simulink model "Startbrenner_Funktionsblock"  (R2019b)
settings: Solver=VariableStepAuto  StartTime=0.0  StopTime=3000  RelTol=1e-3
values from neighbouring files (symbols this model uses):
  A = double(subs(subs(subs( jacobian(dx_dt,vec_x), vec_x, x_AP), vec_e, e_AP), vec_u, u_AP))    [Modellbildung_Startbrenner.m]
  B = double(subs(subs(subs( jacobian(dx_dt,vec_u), vec_x, x_AP), vec_e, e_AP), vec_u, u_AP))    [Modellbildung_Startbrenner.m]
  C = [1,0,0;0,1,0]    [Modellbildung_Startbrenner.m]
  E = double(subs(subs(subs( jacobian(dx_dt,vec_e), vec_x, x_AP), vec_e, e_AP), vec_u, u_AP))    [Modellbildung_Startbrenner.m]
  e_AP = [T_bg_in ; T_wt_in ; T_u]    [Modellbildung_Startbrenner.m]
  K = place(A,B,lambda_w)    [Modellbildung_Startbrenner.m]
  S_v = inv(C*(inv(-A+B*K))*B)    [Modellbildung_Startbrenner.m]
  T_Ini = [ 293.15  ; 293.15 ; 293.15  ]    [Modellbildung_Startbrenner.m]
  T_Ini_Lin = T_Ini - x_AP    [Modellbildung_Startbrenner.m]
  u_AP = [ m_sbg ; m_sair ]    [Modellbildung_Startbrenner.m]
  vec_par = zeros(17,1)    [Modellbildung_Startbrenner.m]
  vec_z = vec_T + e_AP    [Modellbildung_Startbrenner.m]
  w = [1200; 1000]    [Modellbildung_Startbrenner.m]
  x_AP = [double(x_AP_berechnet.x1) ; double(x_AP_berechnet.x2) ; double(x_AP_berechnet.x3)]    [Modellbildung_Startbrenner.m]
  y_AP = [double(x_AP_berechnet.x1) ; double(x_AP_berechnet.x2) ]    [Modellbildung_Startbrenner.m]
libraries: simulink x2
settings Model: Creator=mh981  LastModifiedBy=michael
settings DataIOCC: ReturnWorkspaceOutputs=off
settings DebuggingCC: ArithmeticOperatorsInVariantConditions=warning
settings SFSimCC: CustomCodeUndefinedFunction=UseInterfaceOnly

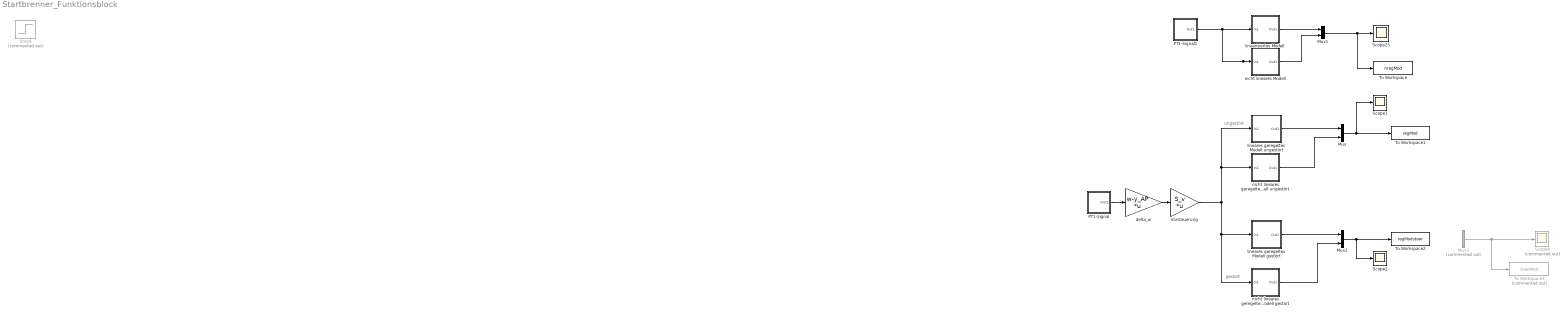
== system Startbrenner_Funktionsblock ==
  note: ungestört
  note: gestört
  Mux : Mux  Inputs=2
  Mux1 : Mux  Inputs=2
  Mux2 : Mux  Inputs=2
  Mux3 : Mux  Commented=on  Inputs=2
  PT1-Signal : Subsystem
  PT1-Signal1 : Subsystem
  Scope1 : Scope
  Scope2 : Scope
  Scope25 : Scope
  Scope4 : Scope  Commented=on
  Step4 : Step  Commented=on  Time=0  Before=u_AP  After=u_AP  SampleTime=0
  To Workspace : ToWorkspace  VariableName=nregMod  SaveFormat=Structure With Time  SampleTime=-1
  To Workspace1 : ToWorkspace  VariableName=regMod  SaveFormat=Structure With Time  SampleTime=-1
  To Workspace2 : ToWorkspace  VariableName=regModstoer  SaveFormat=Structure With Time  SampleTime=-1
  To Workspace3 : ToWorkspace  Commented=on  VariableName=stoerMod  SaveFormat=Structure With Time  SampleTime=-1
  Vorsteuerung : Gain  Gain=S_v  Multiplication=Matrix(K*u)
  delta_w : Gain  Gain=w-y_AP  Multiplication=Matrix(K*u)
  lineares geregeltes Modell gestört : Subsystem
  lineares geregeltes Modell ungestört : Subsystem
  linearisiertes Modell : Subsystem
  nicht lineares Modell : Subsystem
  nicht lineares geregeltes Modell gestört : Subsystem
  nicht lineares geregeltes Modell ungestört : Subsystem
  wires:
  PT1-Signal/1(Out1) -> delta_w/1
  delta_w/1 -> Vorsteuerung/1
  linearisiertes Modell/1(Out1) -> Mux1/1
  PT1-Signal1/1(Out1) -> linearisiertes Modell/1(In1), nicht lineares Modell/1(In1)
  Vorsteuerung/1 -> nicht lineares geregeltes Modell gestört/1(In1), lineares geregeltes Modell gestört/1(In1), lineares geregeltes Modell ungestört/1(In1), nicht lineares geregeltes Modell ungestört/1(In1)
  nicht lineares geregeltes Modell ungestört/1(Out1) -> Mux/2
  lineares geregeltes Modell ungestört/1(Out1) -> Mux/1
  nicht lineares Modell/1(Out1) -> Mux1/2
  Mux/1 -> To Workspace1/1, Scope1/1
  Mux1/1 -> Scope25/1, To Workspace/1
  Mux2/1 -> Scope2/1, To Workspace2/1
  lineares geregeltes Modell gestört/1(Out1) -> Mux2/1
  nicht lineares geregeltes Modell gestört/1(Out1) -> Mux2/2
  Mux3/1 -> To Workspace3/1, Scope4/1

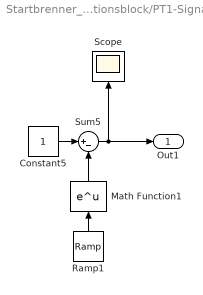
== system Startbrenner_Funktionsblock/PT1-Signal ==
  Constant5 : Constant
  Math Function1 : Math  SignedPower=off  SaturateOnIntegerOverflow=on
  Ramp1 : simulink/Sources/Ramp  slope=-1/t  start=0  InitialOutput=0
  Scope : Scope
  Sum5 : Sum  Inputs=|+-
  Out1 : Outport
  wires:
  Constant5/1 -> Sum5/1
  Math Function1/1 -> Sum5/2
  Ramp1/1 -> Math Function1/1
  Sum5/1 -> Out1/1, Scope/1

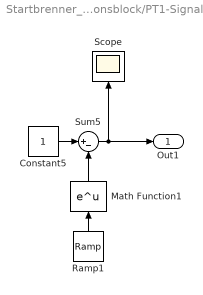
== system Startbrenner_Funktionsblock/PT1-Signal1 ==
  Constant5 : Constant
  Math Function1 : Math  SignedPower=off  SaturateOnIntegerOverflow=on
  Ramp1 : simulink/Sources/Ramp  slope=-1/t  start=0  InitialOutput=0
  Scope : Scope
  Sum5 : Sum  Inputs=|+-
  Out1 : Outport
  wires:
  Constant5/1 -> Sum5/1
  Math Function1/1 -> Sum5/2
  Ramp1/1 -> Math Function1/1
  Sum5/1 -> Out1/1, Scope/1

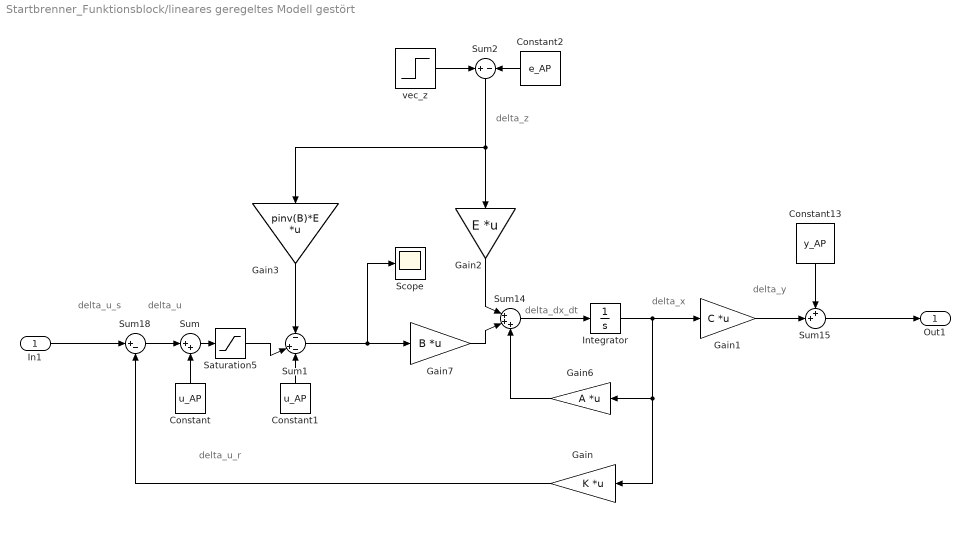
== system Startbrenner_Funktionsblock/lineares geregeltes Modell gestört ==
  note: delta_y
  note: delta_x
  note: delta_dx_dt
  note: delta_u_r
  note: delta_u
  note: delta_u_s
  note: delta_z
  In1 : Inport
  Constant : Constant  Value=u_AP
  Constant1 : Constant  Value=u_AP
  Constant13 : Constant  Value=y_AP
  Constant2 : Constant  Value=e_AP
  Gain : Gain  Gain=K  Multiplication=Matrix(K*u)
  Gain1 : Gain  Gain=C  Multiplication=Matrix(K*u)
  Gain2 : Gain  Gain=E  Multiplication=Matrix(K*u)
  Gain3 : Gain  Gain=pinv(B)*E  Multiplication=Matrix(K*u)
  Gain6 : Gain  Gain=A  Multiplication=Matrix(K*u)
  Gain7 : Gain  Gain=B  Multiplication=Matrix(K*u) (u vector)
  Integrator : Integrator  InitialCondition=T_Ini_Lin
  Saturation5 : Saturate  UpperLimit=2*u_AP  LowerLimit=0.1*u_AP
  Scope : Scope
  Sum : Sum  Inputs=|++
  Sum1 : Sum  Inputs=-|+-
  Sum14 : Sum  Inputs=|+++
  Sum15 : Sum  Inputs=++|
  Sum18 : Sum  Inputs=|+-
  Sum2 : Sum  Inputs=+|-
  vec_z : Step  Before=vec_z  After=vec_z  SampleTime=0
  Out1 : Outport
  wires:
  Gain1/1 -> Sum15/2
  Sum14/1 -> Integrator/1
  vec_z/1 -> Sum2/1
  Sum18/1 -> Sum/1
  Constant1/1 -> Sum1/3
  Gain/1 -> Sum18/2
  Gain2/1 -> Sum14/1
  Saturation5/1 -> Sum1/2
  Constant/1 -> Sum/2
  Sum15/1 -> Out1/1
  Gain6/1 -> Sum14/3
  Constant2/1 -> Sum2/2
  In1/1 -> Sum18/1
  Integrator/1 -> Gain6/1, Gain/1, Gain1/1
  Constant13/1 -> Sum15/1
  Sum/1 -> Saturation5/1
  Sum2/1 -> Gain3/1, Gain2/1
  Gain7/1 -> Sum14/2
  Gain3/1 -> Sum1/1
  Sum1/1 -> Scope/1, Gain7/1

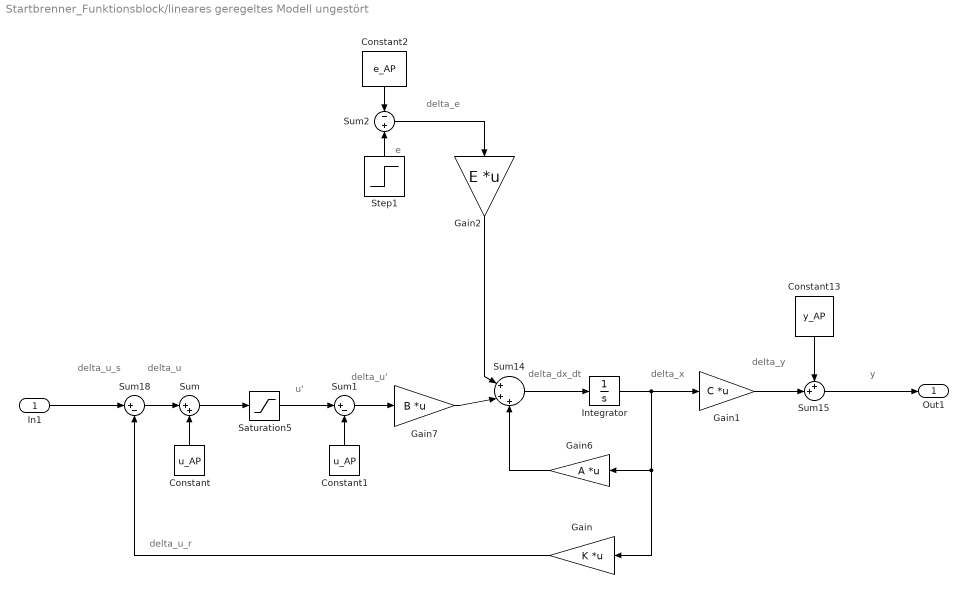
== system Startbrenner_Funktionsblock/lineares geregeltes Modell ungestört ==
  note: delta_u'
  note: u'
  note: y
  note: e
  note: delta_y
  note: delta_x
  note: delta_dx_dt
  note: delta_u_r
  note: delta_u
  note: delta_u_s
  note: delta_e
  In1 : Inport
  Constant : Constant  Value=u_AP
  Constant1 : Constant  Value=u_AP
  Constant13 : Constant  Value=y_AP
  Constant2 : Constant  Value=e_AP
  Gain : Gain  Gain=K  Multiplication=Matrix(K*u)
  Gain1 : Gain  Gain=C  Multiplication=Matrix(K*u)
  Gain2 : Gain  Gain=E  Multiplication=Matrix(K*u)
  Gain6 : Gain  Gain=A  Multiplication=Matrix(K*u)
  Gain7 : Gain  Gain=B  Multiplication=Matrix(K*u) (u vector)
  Integrator : Integrator  InitialCondition=T_Ini_Lin
  Saturation5 : Saturate  UpperLimit=2*u_AP  LowerLimit=0.1*u_AP
  Step1 : Step  Before=e_AP  After=e_AP  SampleTime=0
  Sum : Sum  Inputs=|++
  Sum1 : Sum  Inputs=|+-
  Sum14 : Sum  Inputs=|+++
  Sum15 : Sum  Inputs=++|
  Sum18 : Sum  Inputs=|+-
  Sum2 : Sum  Inputs=-|+
  Out1 : Outport
  wires:
  Gain1/1 -> Sum15/2
  Sum14/1 -> Integrator/1
  Step1/1 -> Sum2/2
  Sum18/1 -> Sum/1
  Constant1/1 -> Sum1/2
  Gain/1 -> Sum18/2
  Gain2/1 -> Sum14/1
  Saturation5/1 -> Sum1/1
  Constant/1 -> Sum/2
  Sum15/1 -> Out1/1
  Gain6/1 -> Sum14/3
  Constant2/1 -> Sum2/1
  Gain7/1 -> Sum14/2
  In1/1 -> Sum18/1
  Integrator/1 -> Gain6/1, Gain/1, Gain1/1
  Constant13/1 -> Sum15/1
  Sum1/1 -> Gain7/1
  Sum/1 -> Saturation5/1
  Sum2/1 -> Gain2/1

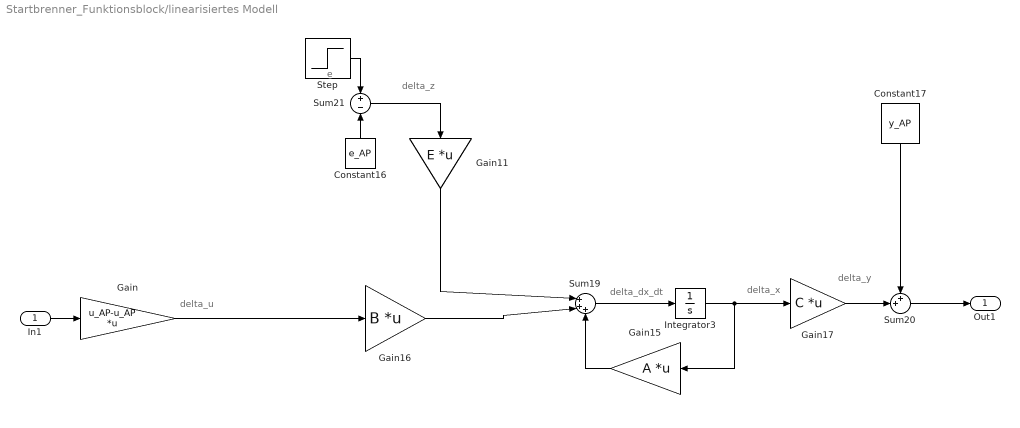
== system Startbrenner_Funktionsblock/linearisiertes Modell ==
  note: delta_dx_dt
  note: delta_x
  note: delta_u
  note: delta_y
  note: e
  note: delta_z
  In1 : Inport
  Constant16 : Constant  Value=e_AP
  Constant17 : Constant  Value=y_AP
  Gain : Gain  Gain=u_AP-u_AP  Multiplication=Matrix(K*u)
  Gain11 : Gain  Gain=E  Multiplication=Matrix(K*u) (u vector)
  Gain15 : Gain  Gain=A  Multiplication=Matrix(K*u) (u vector)
  Gain16 : Gain  Gain=B  Multiplication=Matrix(K*u) (u vector)
  Gain17 : Gain  Gain=C  Multiplication=Matrix(K*u) (u vector)
  Integrator3 : Integrator  InitialCondition=T_Ini_Lin
  Step : Step  Before=e_AP  After=e_AP  SampleTime=0
  Sum19 : Sum  Inputs=|+++
  Sum20 : Sum  Inputs=++|
  Sum21 : Sum  Inputs=+|-
  Out1 : Outport
  wires:
  Sum19/1 -> Integrator3/1
  Gain11/1 -> Sum19/1
  Gain15/1 -> Sum19/3
  Gain16/1 -> Sum19/2
  Sum20/1 -> Out1/1
  In1/1 -> Gain/1
  Constant17/1 -> Sum20/1
  Gain17/1 -> Sum20/2
  Integrator3/1 -> Gain15/1, Gain17/1
  Gain/1 -> Gain16/1
  Sum21/1 -> Gain11/1
  Step/1 -> Sum21/1
  Constant16/1 -> Sum21/2

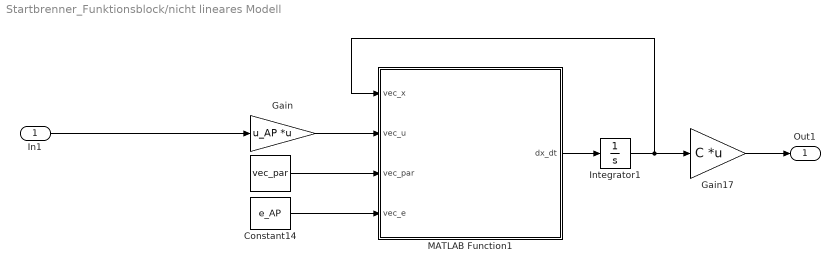
== system Startbrenner_Funktionsblock/nicht lineares Modell ==
  In1 : Inport
  " " : Constant  Value=vec_par
  Constant14 : Constant  Value=e_AP
  Gain : Gain  Gain=u_AP  Multiplication=Matrix(K*u)
  Gain17 : Gain  Gain=C  Multiplication=Matrix(K*u) (u vector)
  Integrator1 : Integrator  InitialCondition=T_Ini
  MATLAB Function1 : MATLAB Function  TreatAsAtomicUnit=on
  Out1 : Outport
  wires:
  In1/1 -> Gain/1
  " "/1 -> MATLAB Function1/3(vec_par)
  Integrator1/1 -> MATLAB Function1/1(vec_x), Gain17/1
  MATLAB Function1/1(dx_dt) -> Integrator1/1
  Gain/1 -> MATLAB Function1/2(vec_u)
  Gain17/1 -> Out1/1
  Constant14/1 -> MATLAB Function1/4(vec_e)

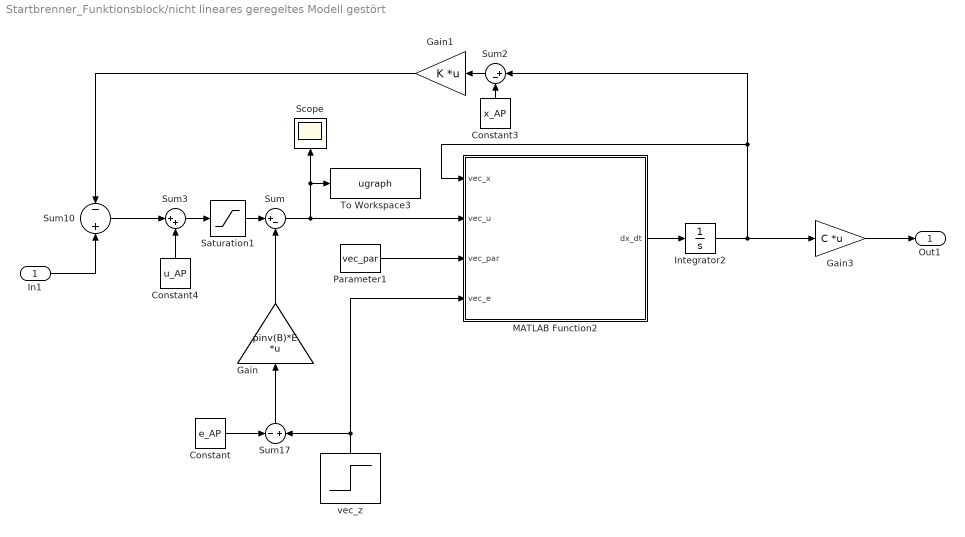
== system Startbrenner_Funktionsblock/nicht lineares geregeltes Modell gestört ==
  In1 : Inport
  Constant : Constant  Value=e_AP
  Constant3 : Constant  Value=x_AP
  Constant4 : Constant  Value=u_AP
  Gain : Gain  Gain=pinv(B)*E  Multiplication=Matrix(K*u)
  Gain1 : Gain  Gain=K  Multiplication=Matrix(K*u) (u vector)
  Gain3 : Gain  Gain=C  Multiplication=Matrix(K*u)
  Integrator2 : Integrator  InitialCondition=T_Ini
  MATLAB Function2 : MATLAB Function  TreatAsAtomicUnit=on
  Parameter1 : Constant  Value=vec_par
  Saturation1 : Saturate  UpperLimit=2*u_AP  LowerLimit=0.1*u_AP
  Scope : Scope
  Sum : Sum  Inputs=|+-
  Sum10 : Sum  Inputs=-|+
  Sum17 : Sum  Inputs=-|+
  Sum2 : Sum  Inputs=|+-
  Sum3 : Sum  Inputs=|++
  To Workspace3 : ToWorkspace  VariableName=ugraph  SaveFormat=Structure With Time  SampleTime=-1
  vec_z : Step  Before=vec_z  After=vec_z  SampleTime=0
  Out1 : Outport
  wires:
  MATLAB Function2/1(dx_dt) -> Integrator2/1
  Gain1/1 -> Sum10/1
  Sum10/1 -> Sum3/1
  Parameter1/1 -> MATLAB Function2/3(vec_par)
  vec_z/1 -> Sum17/2, MATLAB Function2/4(vec_e)
  Gain3/1 -> Out1/1
  Saturation1/1 -> Sum/1
  Sum3/1 -> Saturation1/1
  In1/1 -> Sum10/2
  Constant4/1 -> Sum3/2
  Gain/1 -> Sum/2
  Sum/1 -> MATLAB Function2/2(vec_u), Scope/1, To Workspace3/1
  Constant/1 -> Sum17/1
  Sum17/1 -> Gain/1
  Constant3/1 -> Sum2/2
  Sum2/1 -> Gain1/1
  Integrator2/1 -> Gain3/1, Sum2/1, MATLAB Function2/1(vec_x)

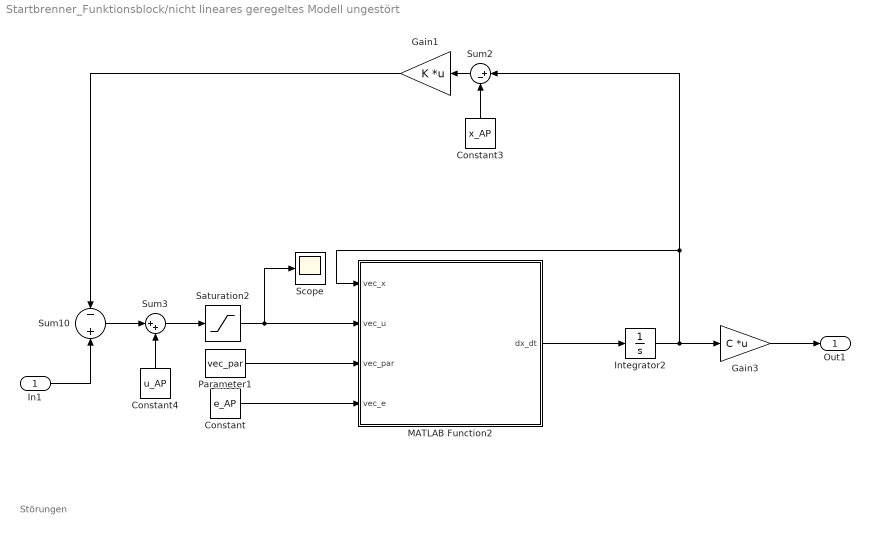
== system Startbrenner_Funktionsblock/nicht lineares geregeltes Modell ungestört ==
  note: Störungen
  In1 : Inport
  Constant : Constant  Value=e_AP
  Constant3 : Constant  Value=x_AP
  Constant4 : Constant  Value=u_AP
  Gain1 : Gain  Gain=K  Multiplication=Matrix(K*u) (u vector)
  Gain3 : Gain  Gain=C  Multiplication=Matrix(K*u)
  Integrator2 : Integrator  InitialCondition=T_Ini
  MATLAB Function2 : MATLAB Function  TreatAsAtomicUnit=on
  Parameter1 : Constant  Value=vec_par
  Saturation2 : Saturate  UpperLimit=2*u_AP  LowerLimit=0.1*u_AP
  Scope : Scope
  Sum10 : Sum  Inputs=-|+
  Sum2 : Sum  Inputs=|+-
  Sum3 : Sum  Inputs=|++
  Out1 : Outport
  wires:
  MATLAB Function2/1(dx_dt) -> Integrator2/1
  Gain1/1 -> Sum10/1
  Sum10/1 -> Sum3/1
  Parameter1/1 -> MATLAB Function2/3(vec_par)
  Gain3/1 -> Out1/1
  Sum3/1 -> Saturation2/1
  In1/1 -> Sum10/2
  Constant4/1 -> Sum3/2
  Saturation2/1 -> Scope/1, MATLAB Function2/2(vec_u)
  Constant/1 -> MATLAB Function2/4(vec_e)
  Constant3/1 -> Sum2/2
  Sum2/1 -> Gain1/1
  Integrator2/1 -> Sum2/1, MATLAB Function2/1(vec_x), Gain3/1

== matlab function Startbrenner_Funktionsblock/nicht lineares Modell/MATLAB Function1 ==
  data: vec_x input; vec_u input; dx_dt output; vec_par input; vec_e input
%#eml
function dx_dt = Modell_simulink(vec_x ,vec_u , vec_par , vec_e)

dx_dt = Modellgleichung_Startbrenner (vec_x ,vec_u , vec_par , vec_e);

== matlab function Startbrenner_Funktionsblock/nicht lineares geregeltes Modell gestört/MATLAB Function2 ==
  data: vec_x input; vec_u input; dx_dt output; vec_par input; vec_e input
%#eml
function dx_dt = Modell_simulink(vec_x ,vec_u , vec_par , vec_e)

dx_dt = Modellgleichung_Startbrenner (vec_x ,vec_u , vec_par , vec_e);

== matlab function Startbrenner_Funktionsblock/nicht lineares geregeltes Modell ungestört/MATLAB Function2 ==
  data: vec_x input; vec_u input; dx_dt output; vec_par input; vec_e input
%#eml
function dx_dt = Modell_simulink(vec_x ,vec_u , vec_par , vec_e)

dx_dt = Modellgleichung_Startbrenner (vec_x ,vec_u , vec_par , vec_e);
